simulink model "quad_sim"  (R2023b)
settings: Solver=ode1  StartTime=0.0  StopTime=100  FixedStep=0.001  RelTol=1e-3
libraries: uavutilslib x1
settings Model: Creator=soemt  LastModifiedBy=soemt

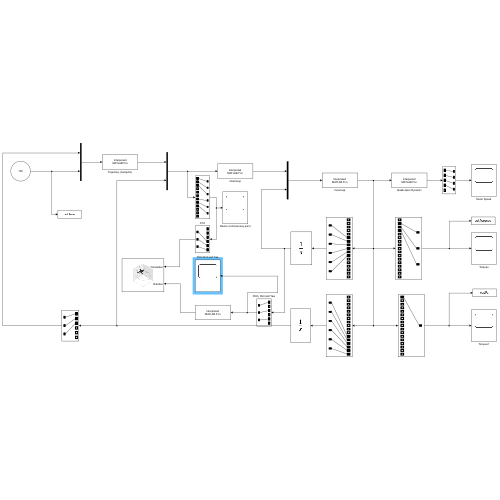
[thumbnail: Simulink's stored preview of the top-level diagram]
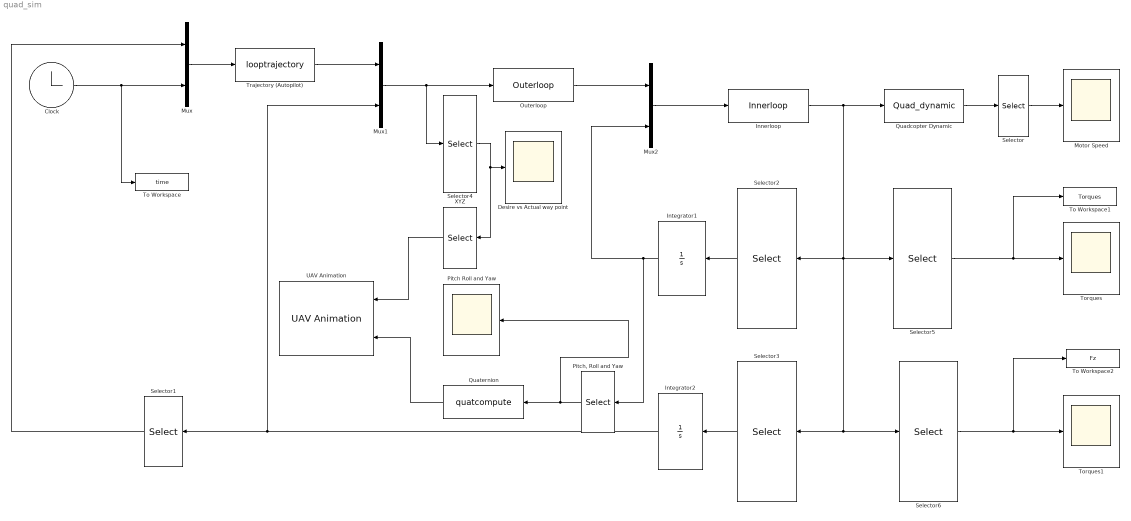
== system quad_sim ==
  Clock : Clock
  Desire vs Actual way point : Scope
  Innerloop : MATLABFcn  MATLABFcn=Innerloop  OutputDimensions=17
  Integrator1 : Integrator  InitialCondition=[0 0 0 0 0 0]
  Integrator2 : Integrator  InitialCondition=[0 0 0 0 0 0]
  Motor Speed : Scope
  Mux : Mux  Inputs=2
  Mux1 : Mux  Inputs=2
  Mux2 : Mux  Inputs=2
  Outerloop : MATLABFcn  MATLABFcn=Outerloop  OutputDimensions=13
  Pitch Roll and Yaw : Scope
  "Pitch, Roll and Yaw" : Selector  InputPortWidth=6  IndexOptions=Index vector (dialog)  Indices=[1 3 5]  OutputSizes=1
  Quadcopter Dynamic : MATLABFcn  MATLABFcn=Quad_dynamic  OutputDimensions=5
  Quaternion : MATLABFcn  MATLABFcn=quatcompute  OutputDimensions=4
  Selector : Selector  InputPortWidth=5  IndexOptions=Index vector (dialog)  Indices=[1 2 3 4]  OutputSizes=1
  Selector1 : Selector  InputPortWidth=6  IndexOptions=Index vector (dialog)  Indices=[1 2 3]  OutputSizes=1
  Selector2 : Selector  InputPortWidth=17  IndexOptions=Index vector (dialog)  Indices=[6 7 8 9 10 11]  OutputSizes=1
  Selector3 : Selector  InputPortWidth=17  IndexOptions=Index vector (dialog)  Indices=[12 13 14 15 16 17]  OutputSizes=1
  Selector4 : Selector  InputPortWidth=12  IndexOptions=Index vector (dialog)  Indices=[1 2 3 7 8 9]  OutputSizes=1
  Selector5 : Selector  InputPortWidth=17  IndexOptions=Index vector (dialog)  Indices=[2 3 4]  OutputSizes=1
  Selector6 : Selector  InputPortWidth=17  IndexOptions=Index vector (dialog)  Indices=[1]  OutputSizes=1
  To Workspace : ToWorkspace  VariableName=time  SampleTime=-1
  To Workspace1 : ToWorkspace  VariableName=Torques  SampleTime=-1
  To Workspace2 : ToWorkspace  VariableName=Fz  SampleTime=-1
  Torques : Scope
  Torques1 : Scope
  Trajectory (Autopilot) : MATLABFcn  MATLABFcn=looptrajectory  OutputDimensions=6
  UAV Animation : uavutilslib/UAV Animation  UAVType=Multirotor  UAVSize=1  InertialZDirection=Up  SampleTime=-1
  XYZ : Selector  InputPortWidth=6  IndexOptions=Index vector (dialog)  Indices=[4 5 6]  OutputSizes=1
  wires:
  Clock/1 -> Mux/2, To Workspace/1
  Mux/1 -> Trajectory (Autopilot)/1
  Trajectory (Autopilot)/1 -> Mux1/1
  Mux1/1 -> Selector4/1, Outerloop/1
  Outerloop/1 -> Mux2/1
  Mux2/1 -> Innerloop/1
  Innerloop/1 -> Selector5/1, Selector6/1, Selector3/1, Selector2/1, Quadcopter Dynamic/1
  Selector2/1 -> Integrator1/1
  Integrator1/1 -> "Pitch, Roll and Yaw"/1, Mux2/2
  Selector3/1 -> Integrator2/1
  Integrator2/1 -> Mux1/2, Selector1/1
  Selector1/1 -> Mux/1
  Quadcopter Dynamic/1 -> Selector/1
  Selector/1 -> Motor Speed/1
  Selector4/1 -> XYZ/1, Desire vs Actual way point/1
  Selector5/1 -> To Workspace1/1, Torques/1
  XYZ/1 -> UAV Animation/1
  Quaternion/1 -> UAV Animation/2
  Selector6/1 -> To Workspace2/1, Torques1/1
  "Pitch, Roll and Yaw"/1 -> Pitch Roll and Yaw/1, Quaternion/1
